simulink model "stm32f4_target_udpcam_demo"  (Simulink 7.3)
settings: Solver=FixedStepDiscrete  SolverMode=SingleTasking  StartTime=0.0  StopTime=1  RelTol=1e-3
PreLoadFcn:
  | waijung.modelPreload; % Required for working with Waijung Blockset. Do not remove.
undefined symbols (not defined in the file): A1, A2, A7, B10, B11, B12, C1, C2, C3, C4, C5, G14, H2, H3, H6, H7, HSEOSC, Link, LQFP176, ST, STM32F417IG
libraries: simulink x11, stm32f4_i2c_lib x8, stm32f4_tim_lib x2, waijung_webserver x2, stm32f4_rcc_lib x1, stm32f4_device_config_lib x1, waijung_socket_lib x1, waijung_addon_module x1
(part 2 of 2)

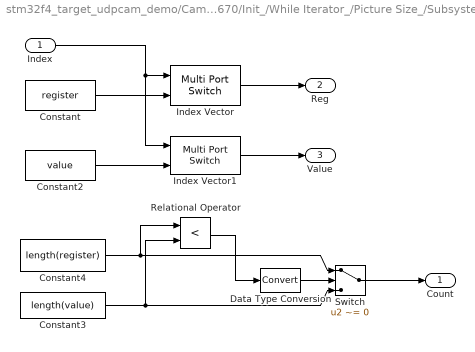
== system stm32f4_target_udpcam_demo/Camera OV7670/Init_/While Iterator_/Picture Size_/Subsystem/Subsystem/Img480x640/Register List ==
  Index : Inport  OutDataType=fixdt(1, 16)  OutScaling=2^0
  Constant : Constant  Value=register  OutDataType=fixdt(1, 16)  OutScaling=2^0
  Constant2 : Constant  Value=value  OutDataType=fixdt(1, 16)  OutScaling=2^0
  Constant3 : Constant  Value=length(value)  OutDataType=fixdt(1, 16)  OutScaling=2^0
  Constant4 : Constant  Value=length(register)  OutDataType=fixdt(1, 16)  OutScaling=2^0
  Data Type Conversion : DataTypeConversion  OutDataType=fixdt(1, 16)  OutScaling=2^0
  Index Vector : MultiPortSwitch  Inputs=1  zeroidx=on  OutDataType=fixdt(1, 16)  OutScaling=2^0
  Index Vector1 : MultiPortSwitch  Inputs=1  zeroidx=on  OutDataType=fixdt(1, 16)  OutScaling=2^0
  Relational Operator : RelationalOperator  Operator=<  LogicOutDataTypeMode=boolean  LogicDataType=fixdt(0, 8)  OutDataTypeStr=boolean
  Switch : Switch  Criteria=u2 ~= 0  OutDataType=fixdt(1, 16)  OutScaling=2^0
  Count : Outport  OutDataType=fixdt(1, 16)  OutScaling=2^0
  Reg : Outport  Port=2  OutDataType=fixdt(1, 16)  OutScaling=2^0
  Value : Outport  Port=3  OutDataType=fixdt(1, 16)  OutScaling=2^0
  wires:
  Index Vector/1 -> Reg/1
  Constant/1 -> Index Vector/2
  Index/1 -> Index Vector/1, Index Vector1/1
  Constant2/1 -> Index Vector1/2
  Index Vector1/1 -> Value/1
  Constant4/1 -> Relational Operator/1, Switch/1
  Constant3/1 -> Relational Operator/2, Switch/3
  Relational Operator/1 -> Data Type Conversion/1
  Switch/1 -> Count/1
  Data Type Conversion/1 -> Switch/2
